simulink model "PubIfDecisionLSM_MDL"  (R2020b)
settings: configuration reference "DspaceConfig" (kept outside this file)
PostLoadFcn:
  | if any(exist('dsrtsu_mdlpostloadfcn', 'file') ~= 0), dsrtsu_mdlpostloadfcn('Execute', bdroot); end
InitFcn:
  | , if any(exist('rtifpga_mdlclblib', 'file') ~= 0), rtifpga_mdlclblib('Init', bdroot); end,
  | , if any(exist('dsmpb_private', 'file') ~= 0), dsmpb_private('dsmpb_mdlclblib', 'Init', bdroot); end,
values from neighbouring files (symbols this model uses):
  P_LSM_ALC_Enable = 0.0    [LSM_Parameter.sldd]
  P_LSM_AwayEdge_offset = 0.1    [LSM_Parameter.sldd]
  P_LSM_CentValidErr = 1.0    [LSM_Parameter.sldd]
  P_LSM_DOP_C0_EN_Limit = 0.8    [LSM_Parameter.sldd]
  P_LSM_DOP_C0_out_Limit = 2.0    [LSM_Parameter.sldd]
  P_LSM_DOP_C1_EN_Limit : value not decoded    [LSM_Parameter.sldd]
  P_LSM_DOP_C1_out_Limit : value not decoded    [LSM_Parameter.sldd]
  P_LSM_DOP_C1AndC2_Lim_X : value not decoded    [LSM_Parameter.sldd]
  P_LSM_DOP_C2_EN_Limit : value not decoded    [LSM_Parameter.sldd]
  P_LSM_DOP_C2_out_Limit : value not decoded    [LSM_Parameter.sldd]
  P_LSM_DOP_In_Pre2Dop_Dis = 1.0    [LSM_Parameter.sldd]
  P_LSM_DOP_Out_Pre2Dop_Dis = 2.0    [LSM_Parameter.sldd]
  P_LSM_DOP_PreDis_X : value not decoded    [LSM_Parameter.sldd]
  P_LSM_DOP_PreDis_Y : value not decoded    [LSM_Parameter.sldd]
  P_LSM_DOPEnableSW = 1.0    [LSM_Parameter.sldd]
  P_LSM_DOPValid_CheckTime = 0.06    [LSM_Parameter.sldd]
  P_LSM_DoubleLine_Curr2Cent_Dislimit = 0.5    [LSM_Parameter.sldd]
  P_LSM_DoubleLine_Dop2Cent_Dislimit = 0.5    [LSM_Parameter.sldd]
  P_LSM_DoubleLine_DOPOut_C1 : value not decoded    [LSM_Parameter.sldd]
  P_LSM_DoubleLine_Pre2Cent_Dislimit = 1.0    [LSM_Parameter.sldd]
  P_LSM_Error_Limit = 0.5    [LSM_Parameter.sldd]
  P_LSM_IFV2CenterAxis = 0.0    [LSM_Parameter.sldd]
  P_LSM_IFV2RearAxis = 0.0    [LSM_Parameter.sldd]
  P_LSM_Line2Edge_limit = 0.5    [LSM_Parameter.sldd]
  P_LSM_Line_Error = 0.1    [LSM_Parameter.sldd]
  P_LSM_LineSTD_Limit = 0.15    [LSM_Parameter.sldd]
  P_LSM_NOH_Switch = 0.0    [LSM_Parameter.sldd]
  P_LSM_OTL_C0_Factor = 1.0    [LSM_Parameter.sldd]
  P_LSM_OTL_C1_Factor = 0.5    [LSM_Parameter.sldd]
  P_LSM_OTL_C2_Factor = 0.5    [LSM_Parameter.sldd]
  P_LSM_Pre2OnlyLineDis = 5.0    [LSM_Parameter.sldd]
  P_LSM_Pre_t = 0.0    [LSM_Parameter.sldd]
  P_LSM_SingleLine_Cent2Edge_Dislimit = 100.0    [LSM_Parameter.sldd]
  P_LSM_SingleLine_Curr2Cent_Dislimit = 0.2    [LSM_Parameter.sldd]
  P_LSM_SingleLine_Dop2Cent_Dislimit = 0.2    [LSM_Parameter.sldd]
  P_LSM_SingleLine_DOPOut_C1 : value not decoded    [LSM_Parameter.sldd]
  P_LSM_SingleLine_Pre2Cent_Dislimit = 0.5    [LSM_Parameter.sldd]
  P_LSM_TJALimitSpd = 60.0    [LSM_Parameter.sldd]
undefined symbols (not defined in the file or in its folder): P_lCS_IFV2CenterAxis, P_LCS_IFV2RearAxis, P_LSM_EntryEdge_offset, P_LSM_EntryLnChngEnSwitch, P_LSM_EntryVanishDis, P_LSM_LinetLostTime, P_LSM_LineWijCal_C12, P_LSM_LineWijCal_C13, P_LSM_MapValid_ErrorSwitch, P_LSM_PosLineLcFac, P_LSM_SpdLim_Stub_Spd, P_LSM_SpdLim_StubLength, P_LSM_SpdTurnAlarm
libraries: simulink x324, TrueDurationTime x11
(part 23 of 25)

== matlab function PubIfDecisionLSM_MDL/Subsystem1/TargetLineCalc_20ms2/TargetLineCalc/TypeConf1/RoadWidthCalc1 ==
  data: LeftType input uint8 size=1; RightType input uint8 size=1; Cnt1K1 input uint8 size=1; Cnt2K1 input uint8 size=1; LeftEn output boolean size=1; RightEn output boolean size=1; Cnt1 output uint8 size=1; Cnt2 output uint8 size=1
function [LeftEn,RightEn,Cnt1,Cnt2] = Delay(LeftType,RightType,Cnt1K1,Cnt2K1)
Cnt1 = max(Cnt1K1 - uint8(1),uint8(0));
Cnt2 = max(Cnt2K1 - uint8(1),uint8(0));
if LeftType~=2 && LeftType~=4 && LeftType~=6 && LeftType~=20
   Cnt1 = uint8(10); 
end
if RightType~=2 && RightType~=4 && RightType~=6 && RightType~=20
   Cnt2 = uint8(10); 
end

if Cnt1>0
    LeftEn = false;
else
    LeftEn = true;
end

if Cnt2>0
    RightEn = false;
else
    RightEn = true;
end
end

== matlab function PubIfDecisionLSM_MDL/Subsystem1/TargetLineCalc_20ms2/TargetLineCalc/VehStation ==
  data: VisLineConf input uint8; LeftMostLane output boolean; VisLineA0 input single; VisLineType input uint8; VisEdgeConf input uint8; VisEdgeA0 input single; RightMostLane output boolean; VisLineColor input
function [LeftMostLane,RightMostLane] = fcn(VisLineConf,VisLineA0,VisLineType,VisEdgeConf,VisEdgeA0,VisLineColor)
LeftMostLane = false;
RightMostLane = false;
% SingleLane = false;
if (VisLineConf(2)>0&&VisEdgeConf(1)>0&&VisLineType(1)==1&&abs(VisLineA0(2)-VisEdgeA0(1))<5)||VisLineColor(1)==2
    LeftMostLane = true;
elseif (VisLineConf(3)>0&&VisEdgeConf(2)>0&&VisLineType(2)==1&&abs(VisLineA0(3)-VisEdgeA0(2))<5)||VisLineColor(2)==2
    RightMostLane = true;
end

== matlab function PubIfDecisionLSM_MDL/Subsystem1/TargetLineCalc_20ms2/TargetLineCalc/VisLineFilter1 ==
  data: tCycle input single size=1; vRef input; OTLineValid input boolean size=1; aOTL input single size=1; bOTL input single size=1; cOTL input single size=1; dOTL input single size=1; R input single size=1; LineUpdate input boolean size=1; dDeltaX input single size=1; dDeltaY input single size=1; CosOfPsi input single size=1; SinOfPsi input single size=1; LineValidK1 input boolean size=1; A3K1 input single size=1; A2K1 input single size=1; A1K1 input single size=1; A0K1 input single size=1; RangeK1 input single size=1; tLostK1 input single size=1; LineValid output boolean size=1; A3 output single size=1; A2 output single size=1; A1 output single size=1; A0 output single size=1; Range output single size=1; tLost output single size=1
function [LineValid,A3,A2,A1,A0,Range,tLost] = ...
    VisFilter(tCycle,vRef,OTLineValid,aOTL,bOTL,cOTL,dOTL,R,LineUpdate,...
    dDeltaX,dDeltaY,CosOfPsi,SinOfPsi,...
    LineValidK1,A3K1,A2K1,A1K1,A0K1,RangeK1,tLostK1)

if (OTLineValid==true)&&(LineUpdate==true)
    LineValid = true;
    A3 = aOTL;
    A2 = bOTL;
    A1 = cOTL;
    A0 = dOTL;
    Range = R;
%     if Range<RangeK1
%         Range = RangeK1 - vRef*tCycle;
%     end
    tLost = single(0);
else
    tLost = min(tLostK1 + tCycle,single(10));
    if (LineValidK1==true)&&(tLost<1)
        xi = [0;0.25*RangeK1;0.5*RangeK1;RangeK1];
        yi = A3K1*xi.^3 + A2K1*xi.^2 + A1K1*xi + A0K1;
        t_dx = xi-dDeltaX;
        t_dy = yi-dDeltaY;
        TmpX = t_dx*CosOfPsi+t_dy*SinOfPsi;
        TmpY = -t_dx*SinOfPsi+t_dy*CosOfPsi;
        [A3,A2,A1,A0] = pl(TmpX,TmpY);
        LineValid = true;
        Range = RangeK1 - vRef*tCycle;
        if Range<1
            LineValid = false;
        end
    else
        LineValid = false;
        A3 = single(0);
        A2 = single(0);
        A1 = single(0);
        A0 = single(0);
        Range = single(0);
    end
end

== matlab function PubIfDecisionLSM_MDL/Subsystem1/TargetLineCalc_20ms2/TargetLineCalc/VisLineFilter2 ==
  data: P_LSM_LinetLostTime input; tF input single size=1; DevValid output boolean size=4; DevAngle output single size=4; DevDis output single size=4; tCycle input single size=1; VisLineConf input uint8 size=4; VisLineReliable input single; a3 input single size=4; a2 input single size=4; a1 input single size=4; a0 input single size=4; R input single size=4; LineUpdate input boolean size=1; dDeltaX input single size=1; dDeltaY input single size=1; CosOfPsi input single size=1; SinOfPsi input single size=1; vRef input single size=1; Lowlimit input single; RoadWidth input single size=1; LeftLineChange input boolean size=1; RightLineChange input boolean size=1; LineConfK1 input uint8 size=4; LineReliableK1 input single; A3K1 input single size=4; A2K1 input single size=4; A1K1 input single size=4; A0K1 input single size=4; RangeK1 input single size=4; tLostK1 input single size=4; LineConf output uint8 size=4; LineReliable output single; A3 output single size=4; A2 output single size=4; A1 output single size=4; A0 output single size=4; Range output single size=4; tLost output single size=4; Avail_timeK1 input single; Avail_disK1 input single; Avail_time output single; Avail_dis output single; fix_timeK1 input; FaultK1 input; fix_time output; Fault output
    function [DevValid,DevAngle,DevDis,LineConf,LineReliable,A3,A2,A1,A0,Range,tLost,Avail_time,Avail_dis,fix_time,Fault] = ...
    VisFilter(P_LSM_LinetLostTime,tF,tCycle,VisLineConf,VisLineReliable,a3,a2,a1,a0,R,LineUpdate,...
    dDeltaX,dDeltaY,CosOfPsi,SinOfPsi,vRef,Lowlimit,RoadWidth,LeftLineChange,RightLineChange,...
    LineConfK1, LineReliableK1,A3K1,A2K1,A1K1,A0K1,RangeK1,tLostK1,Avail_timeK1,Avail_disK1,fix_timeK1,FaultK1)

LineConf = uint8(zeros(4,1));
LineReliable = single(zeros(4,1));
A3 = single(zeros(4,1));
A2 = single(zeros(4,1));
A1 = single(zeros(4,1));
A0 = single(zeros(4,1));
Range = single(zeros(4,1));
tLost = single(zeros(4,1));

Line_std = single(zeros(4,1));
Avail_time = Avail_timeK1;
Avail_dis = Avail_disK1;
fix_time = fix_timeK1;
Fault = FaultK1;

DevValid = false(4,1);
DevAngle = single(zeros(4,1));
DevDis = single(zeros(4,1));

for i=1:4
    if  (LineUpdate==true)&&(VisLineConf(i)>0)&&VisLineReliable(i)>0.01
        LineConf(i) = VisLineConf(i);
        LineReliable(i) = VisLineReliable(i);
        A3(i) = a3(i);
        A2(i) = a2(i);
        A1(i) = a1(i);
        A0(i) = a0(i);
        Range(i) = R(i);
        if Range(i)<RangeK1(i)
            Range(i) = RangeK1(i) - vRef*tCycle;
        end
        tLost(i) = single(0);
        
        if LineConfK1(i)>0
            DevValid(i) = true;
            t_Dist = max(single(15),vRef*1.8);
            xi = [0.05*t_Dist;0.3*t_Dist;0.6*t_Dist;t_Dist];
            yi = A3K1(i)*xi.^3 + A2K1(i)*xi.^2 + A1K1(i)*xi + A0K1(i);
            t_dx = xi-dDeltaX;
            t_dy = yi-dDeltaY;
            TmpX = t_dx*CosOfPsi+t_dy*SinOfPsi;
            TmpY = -t_dx*SinOfPsi+t_dy*CosOfPsi;
            [t3,t2,t1,t0] = pl(TmpX,TmpY);
            
            DevAngle(i) = 57.3*(atan(A1(i)) - atan(t1));
            DevDis(i) = (A0(i) - t0)/sqrt(A1(i)^2 + single(1));
            
            if (abs(DevAngle(i))<3)&&(abs(DevDis(i))<0.06)
                tFilter = 0.05/tF;
                A3(i) = tFilter*(A3(i) - t3) + t3;
                A2(i) = tFilter*(A2(i) - t2) + t2;
                A1(i) = tFilter*(A1(i) - t1) + t1;
                A0(i) = tFilter*(A0(i) - t0) + t0;
            end
        end
    else
        tLost(i) = min(tLostK1(i) + tCycle,single(10));
        if (LineConfK1(i)>0)&&(tLost(i)<P_LSM_LinetLostTime)&&vRef>1.8
            xi = [0.5*vRef;(0.5*vRef+0.25*RangeK1(i));(0.5*vRef+0.5*RangeK1(i));(0.5*vRef+RangeK1(i))];
            yi = A3K1(i)*xi.^3 + A2K1(i)*xi.^2 + A1K1(i)*xi + A0K1(i);
            t_dx = xi-dDeltaX;
            t_dy = yi-dDeltaY;
            TmpX = t_dx*CosOfPsi+t_dy*SinOfPsi;
            TmpY = -t_dx*SinOfPsi+t_dy*CosOfPsi;
            [A3(i),A2(i),A1(i),A0(i)] = pl(TmpX,TmpY);
            LineConf(i) = LineConfK1(i);
            LineReliable(i) = LineReliableK1(i);
            Range(i) = RangeK1(i) - 0.5*vRef*tCycle;
            if Range(i)<5
                LineConf(i) = uint8(0);
            end
        elseif (LineConfK1(i)>0)&&vRef<=1.8
            xi = [0.5*vRef;(0.5*vRef+0.25*RangeK1(i));(0.5*vRef+0.5*RangeK1(i));(0.5*vRef+RangeK1(i))];
            yi = A3K1(i)*xi.^3 + A2K1(i)*xi.^2 + A1K1(i)*xi + A0K1(i);
            t_dx = xi-dDeltaX;
            t_dy = yi-dDeltaY;
            TmpX = t_dx*CosOfPsi+t_dy*SinOfPsi;
            TmpY = -t_dx*SinOfPsi+t_dy*CosOfPsi;
            [A3(i),A2(i),A1(i),A0(i)] = pl(TmpX,TmpY);
            LineConf(i) = LineConfK1(i);
            LineReliable(i) = LineReliableK1(i);
            Range(i) = max(5,RangeK1(i));
        end
    end
end
%%  车道线校验
if LeftLineChange
    Avail_time = [single(0);Avail_timeK1(1)+tCycle;Avail_timeK1(2)+tCycle;Avail_timeK1(3)+tCycle];
    Avail_dis = [single(0);Avail_disK1(1)+tCycle*vRef;Avail_disK1(2)+tCycle*vRef;Avail_disK1(3)+tCycle*vRef];  
elseif RightLineChange
    Avail_time = [Avail_timeK1(2)+tCycle;Avail_timeK1(3)+tCycle;Avail_timeK1(4)+tCycle;single(0)];
    Avail_dis = [Avail_disK1(2)+tCycle*vRef;Avail_disK1(3)+tCycle*vRef;Avail_disK1(4)+tCycle*vRef;single(0)];
else
    for i = 1:4
        if  LineConf(i)>0
            t_Dist = max(single(15),5*vRef);
            xi = [0.05*t_Dist;0.6*t_Dist;0.8*t_Dist;t_Dist];
            yi = A3K1(i)*xi.^3 + A2K1(i)*xi.^2 + A1K1(i)*xi + A0K1(i);
            t_dx = xi-dDeltaX;
            y = A3(i)*t_dx.^3+A2(i)*t_dx.^2+A1(i)*t_dx+A0(i);
            Error = y - yi;
            Line_std(i) = std(Error);
            if Line_std(i)<Lowlimit
                Avail_time(i) = Avail_timeK1(i)+tCycle;
                Avail_dis(i) = Avail_disK1(i)+tCycle*vRef;
            else
                Avail_time(i) = single(0);
                Avail_dis(i) = single(0);
            end
%             if Avail_time(i)>6&&Avail_dis(i)>60
%                 Fault(i) = false;
%             end
%             if Fault(i)==true
%                 fix_time(i) = fix_timeK1(i)+tCycle;
%                 xi = [0.5*vRef;(0.5*vRef+0.25*RangeK1(i));(0.5*vRef+0.5*RangeK1(i));(0.5*vRef+RangeK1(i))];
%                 yi = A3K1(i)*xi.^3 + A2K1(i)*xi.^2 + A1K1(i)*xi + A0K1(i);
%                 t_dx = xi-dDeltaX;
%                 t_dy = yi-dDeltaY;
%                 TmpX = t_dx*CosOfPsi+t_dy*SinOfPsi;
%                 TmpY = -t_dx*SinOfPsi+t_dy*CosOfPsi;
%                 [A3(i),A2(i),A1(i),A0(i)] = pl(TmpX,TmpY);
%                 LineConf(i) = LineConfK1(i);
%                 LineReliable(i) = LineReliableK1(i);
%                 Range(i) = RangeK1(i) - 0.5*vRef*tCycle;
%                 if Range(i)<10||fix_time(i)>2
%                     LineConf(i) = uint8(0);
%                 end
%             else
%                 fix_time(i) = single(0);
%             end
        elseif LineConf(i)==0
            Avail_time(i) = single(0);
            Avail_dis(i) = single(0);
        end
    end
end
Avail_time = min(Avail_time,single(10));
Avail_dis = min(Avail_dis,single(100));

%%   
%    When occur left-line crossing,if L2 lost,the above line offset
%    algorithm may calculate a new L2 line,but now the new L2 line have
%    became L3 line ,so it lead to L2 line and L3 line are the same
if (LeftLineChange||RightLineChange) && VisLineConf(2)==0                       
    A3(2) = A3(3);
    A2(2) = A2(3);
    A1(2) = A1(3);
    A0(2) = A0(3)+RoadWidth*sqrt(1+A1(3)*A1(3));
    LineConf(2) = LineConf(3);
    LineReliable(2) = LineReliable(3);
    Range(2) = Range(3);
elseif  (LeftLineChange||RightLineChange) && VisLineConf(3)==0
    A3(3) = A3(2);
    A2(3) = A2(2);
    A1(3) = A1(2);
    A0(3) = A0(2)-RoadWidth*sqrt(1+A1(2)*A1(2));
    LineConf(3) = LineConf(2);
    LineReliable(3) = LineReliable(2);
    Range(3) = Range(2);
end

== matlab function PubIfDecisionLSM_MDL/Subsystem1/TargetLineCalc_20ms2/TargetLineCalc/VisLineFilter4 ==
  data: EdgeConf output uint8 size=2; EdgeReliable output single; EdgeA3 output single size=2; EdgeA2 output single size=2; EdgeA1 output single size=2; EdgeA0 output single size=2; tCycle input single size=1; VisEdgeConf input uint8 size=2; VisEdgeReliable input single; a3 input single size=2; a2 input single size=2; a1 input single size=2; a0 input single size=2; R input single size=2; LineUpdate input boolean size=1; dDeltaX input single size=1; dDeltaY input single size=1; CosOfPsi input single size=1; SinOfPsi input single size=1; vRef input single size=1; EdgeConfK1 input uint8 size=2; EdgeReliableK1 input single; EdgeA3K1 input single size=2; EdgeA2K1 input single size=2; EdgeA1K1 input single size=2; EdgeA0K1 input single size=2; EdgeRangeK1 input single size=2; EdgetLostK1 input single size=2; EdgeRange output single size=2; EdgetLost output single size=2; Avail_timeK1 input single; Avail_disK1 input single; Avail_time output single; Avail_dis output single
function [EdgeConf,EdgeReliable,EdgeA3,EdgeA2,EdgeA1,EdgeA0,EdgeRange,EdgetLost,Avail_time,Avail_dis] = ...
    VisFilter(tCycle,VisEdgeConf,VisEdgeReliable,a3,a2,a1,a0,R,LineUpdate,...
    dDeltaX,dDeltaY,CosOfPsi,SinOfPsi,vRef,EdgeConfK1,EdgeReliableK1,EdgeA3K1,...
    EdgeA2K1,EdgeA1K1,EdgeA0K1,EdgeRangeK1,EdgetLostK1,Avail_timeK1,Avail_disK1)

EdgeConf = uint8(zeros(2,1));
EdgeReliable = single(zeros(2,1));
EdgeA3 = single(zeros(2,1));
EdgeA2 = single(zeros(2,1));
EdgeA1 = single(zeros(2,1));
EdgeA0 = single(zeros(2,1));
EdgeRange = single(zeros(2,1));
EdgetLost = single(zeros(2,1));
Line_std = single(zeros(2,1));
Avail_time = Avail_timeK1;
Avail_dis = Avail_disK1;

for i=1:2
    if (VisEdgeConf(i)>0)&&(LineUpdate==true)
        EdgeConf(i) = VisEdgeConf(i);
        EdgeReliable(i) = VisEdgeReliable(i);
        EdgeA3(i) = a3(i);
        EdgeA2(i) = a2(i);
        EdgeA1(i) = a1(i);
        EdgeA0(i) = a0(i);
        EdgeRange(i) = R(i);
        EdgetLost(i) = single(0);
    else
        EdgetLost(i) = min(EdgetLostK1(i) + tCycle,single(10));
        if (EdgeConfK1(i)>0)&&(EdgetLost(i)<0.3)
            xi = [0.5*vRef;(0.5*vRef+0.25*EdgeRangeK1(i));(0.5*vRef+0.5*EdgeRangeK1(i));(0.5*vRef+EdgeRangeK1(i))];
            yi = EdgeA3K1(i)*xi.^3 + EdgeA2K1(i)*xi.^2 + EdgeA1K1(i)*xi + EdgeA0K1(i);
            t_dx = xi-dDeltaX;
            t_dy = yi-dDeltaY;
            TmpX = t_dx*CosOfPsi+t_dy*SinOfPsi;
            TmpY = -t_dx*SinOfPsi+t_dy*CosOfPsi;
            [EdgeA3(i),EdgeA2(i),EdgeA1(i),EdgeA0(i)] = pl(TmpX,TmpY);
            EdgeConf(i) = EdgeConfK1(i);
            EdgeReliable(i) = EdgeReliableK1(i);
            EdgeRange(i) = EdgeRangeK1(i) - 0.25*vRef*tCycle;
            
            if EdgeRange(i)<5
                EdgeConf(i) = uint8(0);
            end
            
        else
            EdgeConf(i) = uint8(0);
            EdgeReliable(i) = single(0);
            EdgeA3(i) = single(0);
            EdgeA2(i) = single(0);
            EdgeA1(i) = single(0);
            EdgeA0(i) = single(0);
            EdgeRange(i) = single(0);
        end
    end
end
%%  边界线校验
for i = 1:2
    if EdgeConf(i)>0
        t_Dist = max(single(15),3*vRef);
        xi = [0.05*t_Dist;0.6*t_Dist;0.8*t_Dist;t_Dist];
        yi = EdgeA3K1(i)*xi.^3 + EdgeA2K1(i)*xi.^2 + EdgeA1K1(i)*xi + EdgeA0K1(i);
        t_dx = xi-dDeltaX;
        y = EdgeA3(i)*t_dx.^3+EdgeA2(i)*t_dx.^2+EdgeA1(i)*t_dx+EdgeA0(i);
        Error = y - yi;
        Line_std(i) = std(Error);
        if Line_std(i)<0.15
            Avail_time(i) = Avail_timeK1(i)+tCycle;
            Avail_dis(i) = Avail_disK1(i)+tCycle*vRef;
        else
            Avail_time(i) = single(0);
            Avail_dis(i) = single(0);
        end
    elseif EdgeConf(i)==0
        Avail_time(i) = single(0);
        Avail_dis(i) = single(0);
    end
end

== matlab function PubIfDecisionLSM_MDL/Subsystem1/TargetLineCalc_20ms2/TargetLineCalc/YBranchRi ==
  data: LineUpdate input boolean size=1; RightOffset_b input boolean size=1; vRef input single size=1; RoadWidth input single size=1; A3 input single size=4; A2 input single size=4; A1 input single size=4; A0 input single size=4; Conf input uint8 size=4; Reliable input; DistK1 input single size=1; YBranch_b output boolean size=1; YBranchRi_b output boolean size=1; Dist output single size=1; DistRiK1 input single size=1; DistRi output single size=1
function [YBranch_b,YBranchRi_b,Dist,DistRi] =...
    fcn(LineUpdate,RightOffset_b,vRef,RoadWidth,A3,A2,A1,A0,Conf,Reliable,DistK1,DistRiK1)
%%  判断本车道40米处是否边宽变窄，或者右侧出现分叉车道
Dist = max(DistK1 - 0.02*vRef,single(0));
DistRi = max(DistRiK1 - 0.02*vRef,single(0));
if RightOffset_b
    Dist = DistRi;
    DistRi = single(0);
end
LConf = uint8(0);
RConf = uint8(0);
RRConf = uint8(0);
LA3 = A3(2);
LA2 = A2(2);
LA1 = A1(2); 
LA0 = A0(2);
if Reliable(2)>=0.9
LConf = Conf(2);
end

RA3 = A3(3);
RA2 = A2(3);
RA1 = A1(3); 
RA0 = A0(3);
if Reliable(3)>=0.9
RConf = Conf(3);
end

RRA3 = A3(4);
RRA2 = A2(4);
RRA1 = A1(4); 
RRA0 = A0(4);
if Reliable(4)>=0.9
RRConf = Conf(4);
end

if (LConf>0)&&(RConf>0)&&(LineUpdate)&&abs(LA2)<0.0005&&abs(RA2)<0.0005
    dy0 = (LA0 - RA0)/sqrt(LA1^2 +single(1));
    dy40L = 64000*LA3 + 1600*LA2 + 40*LA1 + LA0;
    dy40R = 64000*RA3 + 1600*RA2 + 40*RA1 + RA0;
    K40 = 3*LA3*1600 + 2*LA2*40 + LA1;
    dy40 = (dy40L - dy40R)/sqrt(K40^2 +single(1));
    if (dy0 - dy40<-0.5)&&(RoadWidth>2.5)&&(RoadWidth<4.2)
        Dist = single(80);
    end
end

if Dist>0
    YBranch_b = true;
else
    YBranch_b = false;
end

if (RConf>0)&&(RRConf>0)&&(LineUpdate)
    dy0 = (RA0 - RRA0)/sqrt(RA1^2 + single(1));
    dy40L = 64000*RA3 + 1600*RA2 + 40*RA1 + RA0;
    dy40R = 64000*RRA3 + 1600*RRA2 + 40*RRA1 + RRA0;
    K40 = 3*RA3*1600 + 2*RA2*40 + RA1;
    dy40 = (dy40L - dy40R)/sqrt(K40^2 + single(1));
    if (vRef>15)&&(abs(dy0 - dy40)>1.0)&&(RoadWidth>2.5)&&(RoadWidth<4.2)
        DistRi = single(80);
    end
end

if DistRi>0
    YBranchRi_b = true;
else
    YBranchRi_b = false;
end

== matlab function PubIfDecisionLSM_MDL/Subsystem1/TargetLineCalc_20ms/TargetLineCalc/TJA2NOA ==
  data: TJALineValid input boolean size=1; HWALineValid output boolean size=1; TJALineA3 input single size=1; TJALineA2 input single size=1; TJALineA1 input single size=1; TJALineA0 input single size=1; TJALineRange input single size=1; HWALineC3 output single size=1; HWALineC2 output single size=1; HWALineC1 output single size=1; HWALineC0 output single size=1; HWARange output single size=1
function [HWALineValid,HWALineC3,HWALineC2,HWALineC1,HWALineC0,HWARange] =...
    fcn(TJALineValid,TJALineA3,TJALineA2,...
    TJALineA1,TJALineA0,TJALineRange)
HWALineValid = TJALineValid;
HWALineC3 = TJALineA3;
HWALineC2 = TJALineA2;
HWALineC1 = TJALineA1;
HWALineC0 = TJALineA0;
HWARange = TJALineRange;

== matlab function PubIfDecisionLSM_MDL/Subsystem1/TargetLineCalc_20ms/TargetLineCalc/TypeConf/MATLAB Function ==
  data: update input; LeftType output uint8 size=1; LeftType_en input uint8 size=1; LeftDLMType_en input uint8 size=1; LeftDECELType_en input uint8; RightType_en input uint8 size=1; RightDLMType_en input uint8 size=1; RightDECELType_en input uint8; LeftColor_en input uint8; LLeftType_en input uint8; LeftTypeK1 input uint8 size=1; LeftDLMTypeK1 input uint8 size=1; LeftDECELTypeK1 input uint8; RightTypeK1 input uint8 size=1; RightDLMTypeK1 input uint8 size=1; LeftDLMType output uint8 size=1; LeftDECELType output; RightType output uint8 size=1; RightDLMType output uint8 size=1; RightDECELTypeK1 input uint8; RightDECELType output; LeftColor_enK1 input uint8; LLeftType_enK1 input uint8; LeftColor output; LLeftType output
function [LeftType,LeftDLMType,LeftDECELType,RightType,RightDLMType,RightDECELType,LeftColor,LLeftType] = ...
    fcn(update,LeftType_en,LeftDLMType_en,LeftDECELType_en,RightType_en,RightDLMType_en,RightDECELType_en,LeftColor_en,LLeftType_en,...
        LeftTypeK1,LeftDLMTypeK1,LeftDECELTypeK1,RightTypeK1,RightDLMTypeK1,RightDECELTypeK1,LeftColor_enK1,LLeftType_enK1)
if update
    LeftType = LeftType_en;
    LeftDLMType = LeftDLMType_en;
    LeftDECELType = LeftDECELType_en;
    RightType = RightType_en;
    RightDLMType = RightDLMType_en;
    RightDECELType = RightDECELType_en;
    LeftColor = LeftColor_en;
    LLeftType = LLeftType_en;
else
    LeftType = LeftTypeK1;
    LeftDLMType = LeftDLMTypeK1;
    LeftDECELType = LeftDECELTypeK1;
    RightType = RightTypeK1;
    RightDLMType = RightDLMTypeK1;
    RightDECELType = RightDECELTypeK1;
    LeftColor = LeftColor_enK1;
    LLeftType = LLeftType_enK1;
end

== matlab function PubIfDecisionLSM_MDL/Subsystem1/TargetLineCalc_20ms/TargetLineCalc/TypeConf/RoadWidthCalc1 ==
  data: LeftType input uint8 size=1; LeftDLMType input; LeftDECELType input; RightType input uint8 size=1; RightDLMType input; RightDECELType input; Cnt1K1 input uint8 size=1; Cnt2K1 input uint8 size=1; LeftEn output boolean size=1; RightEn output boolean size=1; Cnt1 output uint8 size=1; Cnt2 output uint8 size=1
function [LeftEn,RightEn,Cnt1,Cnt2] = Delay(LeftType,LeftDLMType,LeftDECELType,RightType,RightDLMType,RightDECELType,Cnt1K1,Cnt2K1)
Cnt1 = max(Cnt1K1 - uint8(1),uint8(0));
Cnt2 = max(Cnt2K1 - uint8(1),uint8(0));
if LeftType==1||LeftType==6||(LeftType==3&&(LeftDLMType~=2||LeftDLMType~=4))||(LeftType==5&&(LeftDECELType~=2))
   Cnt1 = uint8(10); 
end
if RightType==1||RightType==6||(RightType==3&&(RightDLMType~=2||RightDLMType~=4))||(RightType==5&&(RightDECELType~=2))
   Cnt2 = uint8(10); 
end

if Cnt1>0
    LeftEn = false;
else
    LeftEn = true;
end

if Cnt2>0
    RightEn = false;
else
    RightEn = true;
end
end

== matlab function PubIfDecisionLSM_MDL/Subsystem1/TargetLineCalc_20ms/TargetLineCalc/TypeConf1/RoadWidthCalc1 ==
  data: LeftType input uint8 size=1; RightType input uint8 size=1; Cnt1K1 input uint8 size=1; Cnt2K1 input uint8 size=1; LeftEn output boolean size=1; RightEn output boolean size=1; Cnt1 output uint8 size=1; Cnt2 output uint8 size=1
function [LeftEn,RightEn,Cnt1,Cnt2] = Delay(LeftType,RightType,Cnt1K1,Cnt2K1)
Cnt1 = max(Cnt1K1 - uint8(1),uint8(0));
Cnt2 = max(Cnt2K1 - uint8(1),uint8(0));
if LeftType~=2 || LeftType~=4 || LeftType~=6
   Cnt1 = uint8(10); 
end
if RightType~=2 || RightType~=4 || RightType~=6
   Cnt2 = uint8(10); 
end

if Cnt1>0
    LeftEn = false;
else
    LeftEn = true;
end

if Cnt2>0
    RightEn = false;
else
    RightEn = true;
end
end

== matlab function PubIfDecisionLSM_MDL/Subsystem1/TargetLineCalc_20ms/TargetLineCalc/VehStation ==
  data: VisLineConf input uint8; LeftMostLane output boolean; VisLineA0 input single; VisLineType input uint8; VisEdgeConf input uint8; VisEdgeA0 input single; RightMostLane output boolean; VisLineColor input
function [LeftMostLane,RightMostLane] = fcn(VisLineConf,VisLineA0,VisLineType,VisEdgeConf,VisEdgeA0,VisLineColor)
LeftMostLane = false;
RightMostLane = false;
% SingleLane = false;
if (VisLineConf(2)>0&&VisEdgeConf(1)>0&&VisLineType(1)==1&&abs(VisLineA0(2)-VisEdgeA0(1))<5)||VisLineColor(1)==2
    LeftMostLane = true;
elseif (VisLineConf(3)>0&&VisEdgeConf(2)>0&&VisLineType(2)==1&&abs(VisLineA0(3)-VisEdgeA0(2))<5)||VisLineColor(2)==2
    RightMostLane = true;
end

== matlab function PubIfDecisionLSM_MDL/Subsystem1/TargetLineCalc_20ms/TargetLineCalc/VisLineFilter1 ==
  data: tCycle input single size=1; vRef input; OTLineValid input boolean size=1; aOTL input single size=1; bOTL input single size=1; cOTL input single size=1; dOTL input single size=1; R input single size=1; LineUpdate input boolean size=1; dDeltaX input single size=1; dDeltaY input single size=1; CosOfPsi input single size=1; SinOfPsi input single size=1; LineValidK1 input boolean size=1; A3K1 input single size=1; A2K1 input single size=1; A1K1 input single size=1; A0K1 input single size=1; RangeK1 input single size=1; tLostK1 input single size=1; LineValid output boolean size=1; A3 output single size=1; A2 output single size=1; A1 output single size=1; A0 output single size=1; Range output single size=1; tLost output single size=1
function [LineValid,A3,A2,A1,A0,Range,tLost] = ...
    VisFilter(tCycle,vRef,OTLineValid,aOTL,bOTL,cOTL,dOTL,R,LineUpdate,...
    dDeltaX,dDeltaY,CosOfPsi,SinOfPsi,...
    LineValidK1,A3K1,A2K1,A1K1,A0K1,RangeK1,tLostK1)

if (OTLineValid==true)&&(LineUpdate==true)
    LineValid = true;
    A3 = aOTL;
    A2 = bOTL;
    A1 = cOTL;
    A0 = dOTL;
    Range = R;
%     if Range<RangeK1
%         Range = RangeK1 - vRef*tCycle;
%     end
    tLost = single(0);
else
    tLost = min(tLostK1 + tCycle,single(10));
    if (LineValidK1==true)&&(tLost<1)&&vRef>1.8
        xi = [0;0.25*RangeK1;0.5*RangeK1;RangeK1];
        yi = A3K1*xi.^3 + A2K1*xi.^2 + A1K1*xi + A0K1;
        t_dx = xi-dDeltaX;
        t_dy = yi-dDeltaY;
        TmpX = t_dx*CosOfPsi+t_dy*SinOfPsi;
        TmpY = -t_dx*SinOfPsi+t_dy*CosOfPsi;
        [A3,A2,A1,A0] = pl(TmpX,TmpY);
        LineValid = true;
        Range = RangeK1 - vRef*tCycle;
        if Range<1
            LineValid = false;
        end
    elseif LineValidK1==true&&vRef<=1.8
         xi = [0;0.25*RangeK1;0.5*RangeK1;RangeK1];
        yi = A3K1*xi.^3 + A2K1*xi.^2 + A1K1*xi + A0K1;
        t_dx = xi-dDeltaX;
        t_dy = yi-dDeltaY;
        TmpX = t_dx*CosOfPsi+t_dy*SinOfPsi;
        TmpY = -t_dx*SinOfPsi+t_dy*CosOfPsi;
        [A3,A2,A1,A0] = pl(TmpX,TmpY);
        LineValid = true;
        Range = max(single(5),RangeK1);
    else
        LineValid = false;
        A3 = single(0);
        A2 = single(0);
        A1 = single(0);
        A0 = single(0);
        Range = single(0);
    end
end

== matlab function PubIfDecisionLSM_MDL/Subsystem1/TargetLineCalc_20ms/TargetLineCalc/VisLineFilter2 ==
  data: tF input single size=1; DevValid output boolean size=4; DevAngle output single size=4; DevDis output single size=4; tCycle input single size=1; VisLineConf input uint8 size=4; VisLineReliable input single; a3 input single size=4; a2 input single size=4; a1 input single size=4; a0 input single size=4; R input single size=4; LineUpdate input boolean size=1; dDeltaX input single size=1; dDeltaY input single size=1; CosOfPsi input single size=1; SinOfPsi input single size=1; vRef input single size=1; Lowlimit input single; RoadWidth input single size=1; LeftLineChange input boolean size=1; RightLineChange input boolean size=1; LH1Wij input single; LH2Wij input single; LineConfK1 input uint8 size=4; LineReliableK1 input single; A3K1 input single size=4; A2K1 input single size=4; A1K1 input single size=4; A0K1 input single size=4; RangeK1 input single size=4; tLostK1 input single size=4; LineConf output uint8 size=4; LineReliable output single; A3 output single size=4; A2 output single size=4; A1 output single size=4; A0 output single size=4; Range output single size=4; tLost output single size=4; Avail_timeK1 input single; Avail_disK1 input single; Avail_time output single; Avail_dis output single; fix_timeK1 input; FaultK1 input; fix_time output; Fault output
    function [DevValid,DevAngle,DevDis,LineConf,LineReliable,A3,A2,A1,A0,Range,tLost,Avail_time,Avail_dis,fix_time,Fault] = ...
    VisFilter(tF,tCycle,VisLineConf,VisLineReliable,a3,a2,a1,a0,R,LineUpdate,...
    dDeltaX,dDeltaY,CosOfPsi,SinOfPsi,vRef,Lowlimit,RoadWidth,LeftLineChange,RightLineChange,LH1Wij,LH2Wij,...
    LineConfK1, LineReliableK1,A3K1,A2K1,A1K1,A0K1,RangeK1,tLostK1,Avail_timeK1,Avail_disK1,fix_timeK1,FaultK1)

LineConf = uint8(zeros(4,1));
LineReliable = single(zeros(4,1));
A3 = single(zeros(4,1));
A2 = single(zeros(4,1));
A1 = single(zeros(4,1));
A0 = single(zeros(4,1));
Range = single(zeros(4,1));
tLost = single(zeros(4,1));

Line_std = single(zeros(4,1));
Avail_time = Avail_timeK1;
Avail_dis = Avail_disK1;
fix_time = fix_timeK1;
Fault = FaultK1;

DevValid = false(4,1);
DevAngle = single(zeros(4,1));
DevDis = single(zeros(4,1));

for i=1:4
    if  (LineUpdate==true)&&(VisLineConf(i)>0)&&VisLineReliable(i)>0.01  
        LineConf(i) = VisLineConf(i);
        LineReliable(i) = VisLineReliable(i);
        A3(i) = a3(i);
        A2(i) = a2(i);
        A1(i) = a1(i);
        A0(i) = a0(i);
        Range(i) = R(i);
        if Range(i)<RangeK1(i)
            Range(i) = RangeK1(i) - vRef*tCycle;
        end
        tLost(i) = single(0);
        
        if LineConfK1(i)>0
            DevValid(i) = true;
            t_Dist = max(single(15),vRef*1.8);
            xi = [0.05*t_Dist;0.3*t_Dist;0.6*t_Dist;t_Dist];
            yi = A3K1(i)*xi.^3 + A2K1(i)*xi.^2 + A1K1(i)*xi + A0K1(i);
            t_dx = xi-dDeltaX;
            t_dy = yi-dDeltaY;
            TmpX = t_dx*CosOfPsi+t_dy*SinOfPsi;
            TmpY = -t_dx*SinOfPsi+t_dy*CosOfPsi;
            [t3,t2,t1,t0] = pl(TmpX,TmpY);
            
            DevAngle(i) = 57.3*(atan(A1(i)) - atan(t1));
            DevDis(i) = (A0(i) - t0)/sqrt(A1(i)^2 + single(1));
            
            if (abs(DevAngle(i))<3)&&(abs(DevDis(i))<0.06)
                tFilter = 0.05/tF;
                A3(i) = tFilter*(A3(i) - t3) + t3;
                A2(i) = tFilter*(A2(i) - t2) + t2;
                A1(i) = tFilter*(A1(i) - t1) + t1;
                A0(i) = tFilter*(A0(i) - t0) + t0;
            end
        end
    else
        tLost(i) = min(tLostK1(i) + tCycle,single(10));
        if (LineConfK1(i)>0)&&(tLost(i)<0.5)&&vRef>1.8
            xi = [0.5*vRef;(0.5*vRef+0.25*RangeK1(i));(0.5*vRef+0.5*RangeK1(i));(0.5*vRef+RangeK1(i))];
            yi = A3K1(i)*xi.^3 + A2K1(i)*xi.^2 + A1K1(i)*xi + A0K1(i);
            t_dx = xi-dDeltaX;
            t_dy = yi-dDeltaY;
            TmpX = t_dx*CosOfPsi+t_dy*SinOfPsi;
            TmpY = -t_dx*SinOfPsi+t_dy*CosOfPsi;
            [A3(i),A2(i),A1(i),A0(i)] = pl(TmpX,TmpY);
            LineConf(i) = LineConfK1(i);
            LineReliable(i) = LineReliableK1(i);
            Range(i) = RangeK1(i) - 0.5*vRef*tCycle;
            if Range(i)<5
                LineConf(i) = uint8(0);
            end
        elseif (LineConfK1(i)>0)&&vRef<=1.8
            xi = [0.5*vRef;(0.5*vRef+0.25*RangeK1(i));(0.5*vRef+0.5*RangeK1(i));(0.5*vRef+RangeK1(i))];
            yi = A3K1(i)*xi.^3 + A2K1(i)*xi.^2 + A1K1(i)*xi + A0K1(i);
            t_dx = xi-dDeltaX;
            t_dy = yi-dDeltaY;
            TmpX = t_dx*CosOfPsi+t_dy*SinOfPsi;
            TmpY = -t_dx*SinOfPsi+t_dy*CosOfPsi;
            [A3(i),A2(i),A1(i),A0(i)] = pl(TmpX,TmpY);
            LineConf(i) = LineConfK1(i);
            LineReliable(i) = LineReliableK1(i);
            Range(i) = max(5,RangeK1(i));
        end
    end
end
%%  车道线校验
if LeftLineChange
    Avail_time = [single(0);Avail_timeK1(1)+tCycle;Avail_timeK1(2)+tCycle;Avail_timeK1(3)+tCycle];
    Avail_dis = [single(0);Avail_disK1(1)+tCycle*vRef;Avail_disK1(2)+tCycle*vRef;Avail_disK1(3)+tCycle*vRef];  
elseif RightLineChange
    Avail_time = [Avail_timeK1(2)+tCycle;Avail_timeK1(3)+tCycle;Avail_timeK1(4)+tCycle;single(0)];
    Avail_dis = [Avail_disK1(2)+tCycle*vRef;Avail_disK1(3)+tCycle*vRef;Avail_disK1(4)+tCycle*vRef;single(0)];
else
    for i = 1:4
        if  LineConf(i)>0
            t_Dist = max(single(15),5*vRef);
            xi = [0.05*t_Dist;0.6*t_Dist;0.8*t_Dist;t_Dist];
            yi = A3K1(i)*xi.^3 + A2K1(i)*xi.^2 + A1K1(i)*xi + A0K1(i);
            t_dx = xi-dDeltaX;
            y = A3(i)*t_dx.^3+A2(i)*t_dx.^2+A1(i)*t_dx+A0(i);
            Error = y - yi;
            Line_std(i) = std(Error);
            if Line_std(i)<Lowlimit
                Avail_time(i) = Avail_timeK1(i)+tCycle;
                Avail_dis(i) = Avail_disK1(i)+tCycle*vRef;
            else
                Avail_time(i) = single(0);
                Avail_dis(i) = single(0);
            end
%             if Avail_time(i)>6&&Avail_dis(i)>60
%                 Fault(i) = false;
%             end
%             if Fault(i)==true
%                 fix_time(i) = fix_timeK1(i)+tCycle;
%                 xi = [0.5*vRef;(0.5*vRef+0.25*RangeK1(i));(0.5*vRef+0.5*RangeK1(i));(0.5*vRef+RangeK1(i))];
%                 yi = A3K1(i)*xi.^3 + A2K1(i)*xi.^2 + A1K1(i)*xi + A0K1(i);
%                 t_dx = xi-dDeltaX;
%                 t_dy = yi-dDeltaY;
%                 TmpX = t_dx*CosOfPsi+t_dy*SinOfPsi;
%                 TmpY = -t_dx*SinOfPsi+t_dy*CosOfPsi;
%                 [A3(i),A2(i),A1(i),A0(i)] = pl(TmpX,TmpY);
%                 LineConf(i) = LineConfK1(i);
%                 LineReliable(i) = LineReliableK1(i);
%                 Range(i) = RangeK1(i) - 0.5*vRef*tCycle;
%                 if Range(i)<10||fix_time(i)>2
%                     LineConf(i) = uint8(0);
%                 end
%             else
%                 fix_time(i) = single(0);
%             end
        elseif LineConf(i)==0
            Avail_time(i) = single(0);
            Avail_dis(i) = single(0);
        end
    end
end
Avail_time = min(Avail_time,single(10));
Avail_dis = min(Avail_dis,single(100));

%%   
%    When occur left-line crossing,if L2 lost,the above line offset
%    algorithm may calculate a new L2 line,but now the new L2 line have
%    became L3 line ,so it lead to L2 line and L3 line are the same
if (LeftLineChange||RightLineChange) && VisLineConf(2)==0                       
    A3(2) = A3(3);
    A2(2) = A2(3);
    A1(2) = A1(3);
    A0(2) = A0(3)+RoadWidth*sqrt(1+A1(3)*A1(3));
    LineConf(2) = LineConf(3);
    LineReliable(2) = LineReliable(3);
    Range(2) = Range(3);
elseif  (LeftLineChange||RightLineChange) && VisLineConf(3)==0
    A3(3) = A3(2);
    A2(3) = A2(2);
    A1(3) = A1(2);
    A0(3) = A0(2)-RoadWidth*sqrt(1+A1(2)*A1(2));
    LineConf(3) = LineConf(2);
    LineReliable(3) = LineReliable(2);
    Range(3) = Range(2);
end

== matlab function PubIfDecisionLSM_MDL/Subsystem1/TargetLineCalc_20ms/TargetLineCalc/VisLineFilter3 ==
  data: DoubleLineLost_b output; LeftOffset_b output boolean; RightOffset_b output boolean; Quality output single; tCycle input single size=1; vRef input; CentLineValid input boolean size=1; CentLineA3 input single size=1; CentLineA2 input single size=1; CentLineA1 input single size=1; CentLineA0 input single; CentLineRange input single; CentQ input single size=1; RoadWidth input; LineUpdate input boolean size=1; dDeltaX input single size=1; dDeltaY input single size=1; CosOfPsi input single size=1; SinOfPsi input single size=1; QualityK1 input single; LineValidK1 input boolean size=1; A3K1 input single size=1; A2K1 input single size=1; A1K1 input single size=1; A0K1 input single size=1; RangeK1 input single size=1; tLostK1 input single size=1; LineValid output boolean size=1; A3 output single size=1; A2 output single size=1; A1 output single size=1; A0 output single size=1; Range output single size=1; tLost output single size=1
function [DoubleLineLost_b,LeftOffset_b,RightOffset_b,Quality,LineValid,A3,A2,A1,A0,Range,tLost] = ...
    VisFilter(tCycle,vRef,CentLineValid,CentLineA3,CentLineA2,CentLineA1,CentLineA0,CentLineRange, CentQ, RoadWidth,LineUpdate,...
    dDeltaX,dDeltaY,CosOfPsi,SinOfPsi,...
    QualityK1,LineValidK1,A3K1,A2K1,A1K1,A0K1,RangeK1,tLostK1)

if (CentLineValid==true)&&(LineUpdate==true)
    LineValid = true;
    A3 = CentLineA3;
    A2 = CentLineA2;
    A1 = CentLineA1;
    A0 = CentLineA0;
    Range = CentLineRange;
    Quality=single(CentQ);
    %     if Range<RangeK1
    %         Range = RangeK1 - vRef*tCycle;
    %     end
    tLost = single(0);
else
    tLost = min(tLostK1 + tCycle,single(10));
    if (LineValidK1==true)&&(tLost<0.5)
        xi = [0;0.25*RangeK1;0.5*RangeK1;RangeK1];
        yi = A3K1*xi.^3 + A2K1*xi.^2 + A1K1*xi + A0K1;
        t_dx = xi-dDeltaX;
        t_dy = yi-dDeltaY;
        TmpX = t_dx*CosOfPsi+t_dy*SinOfPsi;
        TmpY = -t_dx*SinOfPsi+t_dy*CosOfPsi;
        [A3,A2,A1,A0] = pl(TmpX,TmpY);
        LineValid = true;
        Quality=QualityK1;
        Range = RangeK1;
        if Range<5
            LineValid = false;
        end
    else
        LineValid = false;
        A3 = single(0);
        A2 = single(0);
        A1 = single(0);
        A0 = single(0);
        Range = single(0);
        Quality=single(0);
    end
end

if (A0>0)&&(A0K1<0)&&...
        (abs(A0-A0K1)>(RoadWidth - single(1.5)))&&...
        (LineValid==true)&&(LineValidK1==true)
    LeftOffset_b = true;
else
    LeftOffset_b = false;
end
if (A0<0)&&(A0K1>0)&&...
        (abs(A0-A0K1)>(RoadWidth - single(1.5)))&&...
        (LineValid==true)&&(LineValidK1==true)
    RightOffset_b = true;
else
    RightOffset_b = false;
end


if LineValid==false
    DoubleLineLost_b = true;
else
    DoubleLineLost_b = false;
end

== matlab function PubIfDecisionLSM_MDL/Subsystem1/TargetLineCalc_20ms/TargetLineCalc/VisLineFilter4 ==
  data: EdgeConf output uint8 size=2; EdgeReliable output single; EdgeA3 output single size=2; EdgeA2 output single size=2; EdgeA1 output single size=2; EdgeA0 output single size=2; tCycle input single size=1; VisEdgeConf input uint8 size=2; VisEdgeReliable input single; a3 input single size=2; a2 input single size=2; a1 input single size=2; a0 input single size=2; R input single size=2; LineUpdate input boolean size=1; dDeltaX input single size=1; dDeltaY input single size=1; CosOfPsi input single size=1; SinOfPsi input single size=1; vRef input single size=1; EdgeConfK1 input uint8 size=2; EdgeReliableK1 input single; EdgeA3K1 input single size=2; EdgeA2K1 input single size=2; EdgeA1K1 input single size=2; EdgeA0K1 input single size=2; EdgeRangeK1 input single size=2; EdgetLostK1 input single size=2; EdgeRange output single size=2; EdgetLost output single size=2; Avail_timeK1 input single; Avail_disK1 input single; Avail_time output single; Avail_dis output single
function [EdgeConf,EdgeReliable,EdgeA3,EdgeA2,EdgeA1,EdgeA0,EdgeRange,EdgetLost,Avail_time,Avail_dis] = ...
    VisFilter(tCycle,VisEdgeConf,VisEdgeReliable,a3,a2,a1,a0,R,LineUpdate,...
    dDeltaX,dDeltaY,CosOfPsi,SinOfPsi,vRef,EdgeConfK1,EdgeReliableK1,EdgeA3K1,...
    EdgeA2K1,EdgeA1K1,EdgeA0K1,EdgeRangeK1,EdgetLostK1,Avail_timeK1,Avail_disK1)

EdgeConf = uint8(zeros(2,1));
EdgeReliable = single(zeros(2,1));
EdgeA3 = single(zeros(2,1));
EdgeA2 = single(zeros(2,1));
EdgeA1 = single(zeros(2,1));
EdgeA0 = single(zeros(2,1));
EdgeRange = single(zeros(2,1));
EdgetLost = single(zeros(2,1));
Line_std = single(zeros(2,1));
Avail_time = Avail_timeK1;
Avail_dis = Avail_disK1;

for i=1:2
    if (VisEdgeConf(i)>0)&&(LineUpdate==true)
        EdgeConf(i) = VisEdgeConf(i);
        EdgeReliable(i) = VisEdgeReliable(i);
        EdgeA3(i) = a3(i);
        EdgeA2(i) = a2(i);
        EdgeA1(i) = a1(i);
        EdgeA0(i) = a0(i);
        EdgeRange(i) = R(i);
        EdgetLost(i) = single(0);
    else
        EdgetLost(i) = min(EdgetLostK1(i) + tCycle,single(10));
        if (EdgeConfK1(i)>0)&&(EdgetLost(i)<0.3)
            xi = [0.5*vRef;(0.5*vRef+0.25*EdgeRangeK1(i));(0.5*vRef+0.5*EdgeRangeK1(i));(0.5*vRef+EdgeRangeK1(i))];
            yi = EdgeA3K1(i)*xi.^3 + EdgeA2K1(i)*xi.^2 + EdgeA1K1(i)*xi + EdgeA0K1(i);
            t_dx = xi-dDeltaX;
            t_dy = yi-dDeltaY;
            TmpX = t_dx*CosOfPsi+t_dy*SinOfPsi;
            TmpY = -t_dx*SinOfPsi+t_dy*CosOfPsi;
            [EdgeA3(i),EdgeA2(i),EdgeA1(i),EdgeA0(i)] = pl(TmpX,TmpY);
            EdgeConf(i) = EdgeConfK1(i);
            EdgeReliable(i) = EdgeReliableK1(i);
            EdgeRange(i) = EdgeRangeK1(i) - 0.25*vRef*tCycle;
            
            if EdgeRange(i)<5
                EdgeConf(i) = uint8(0);
            end
            
        else
            EdgeConf(i) = uint8(0);
            EdgeReliable(i) = single(0);
            EdgeA3(i) = single(0);
            EdgeA2(i) = single(0);
            EdgeA1(i) = single(0);
            EdgeA0(i) = single(0);
            EdgeRange(i) = single(0);
        end
    end
end
%%  边界线校验
for i = 1:2
    if EdgeConf(i)>0
        t_Dist = max(single(15),3*vRef);
        xi = [0.05*t_Dist;0.6*t_Dist;0.8*t_Dist;t_Dist];
        yi = EdgeA3K1(i)*xi.^3 + EdgeA2K1(i)*xi.^2 + EdgeA1K1(i)*xi + EdgeA0K1(i);
        t_dx = xi-dDeltaX;
        y = EdgeA3(i)*t_dx.^3+EdgeA2(i)*t_dx.^2+EdgeA1(i)*t_dx+EdgeA0(i);
        Error = y - yi;
        Line_std(i) = std(Error);
        if Line_std(i)<0.15
            Avail_time(i) = Avail_timeK1(i)+tCycle;
            Avail_dis(i) = Avail_disK1(i)+tCycle*vRef;
        else
            Avail_time(i) = single(0);
            Avail_dis(i) = single(0);
        end
    elseif EdgeConf(i)==0
        Avail_time(i) = single(0);
        Avail_dis(i) = single(0);
    end
end

== matlab function PubIfDecisionLSM_MDL/Subsystem1/TargetLineCalc_20ms/TargetLineCalc/VisLineFilter5 ==
  data: LeftOffset_b input boolean size=1; RightOffset_b input boolean; LckLock_b input boolean size=1; LckLock_bK1 input boolean size=1; CentLineValid input boolean size=1; CentLineC3 input single size=1; CentLineC2 input single; CentLineC1 input single; CentLineC0 input single; CentLineRange input single; CentLineReliable input single; LeftLineValid input boolean; LeftLineC3 input single; LeftLineC2 input single; LeftLineC1 input single; LeftLineC0 input single; LeftLineRange input single; LeftLineReliable input single; LeftLaneAvail input boolean; RightLineValid input boolean; RightLineC3 input single; RightLineC2 input single; RightLineC1 input single; RightLineC0 input single; RightLineRange input single; RightLineReliable input single; PathValid output boolean; PathA3 output single; PathA2 output single; PathA1 output single; PathA0 output single; PathRange output single; PathReliable output single; RightLaneAvail input boolean; PathLaneAvail output boolean size=3; LockIDK1 input int8; LockID output int8
function [PathValid,PathA3,PathA2,PathA1,PathA0,PathRange,PathReliable,PathLaneAvail,LockID] = ...
    VisFilter(LeftOffset_b,RightOffset_b,LckLock_b,LckLock_bK1,...
    CentLineValid,CentLineC3,CentLineC2,CentLineC1,CentLineC0,CentLineRange,CentLineReliable,...
    LeftLineValid,LeftLineC3,LeftLineC2,LeftLineC1,LeftLineC0,LeftLineRange,LeftLineReliable,LeftLaneAvail,...
    RightLineValid,RightLineC3,RightLineC2,RightLineC1,RightLineC0,RightLineRange,RightLineReliable,RightLaneAvail,LockIDK1)

PathValid = false(3,1);
PathA3 = single(zeros(3,1));
PathA2 = single(zeros(3,1));
PathA1 = single(zeros(3,1));
PathA0 = single(zeros(3,1));
PathRange = single(zeros(3,1));
PathReliable = single(zeros(3,1));
PathLaneAvail = false(3,1);

if LckLock_b
    LockID = LockIDK1;
else
    LockID = int8(0);
end

if (LckLock_b==true)&&(LckLock_bK1==true)
    if LeftOffset_b
        LockID = LockID + int8(1);
    end
    if RightOffset_b
        LockID = LockID + int8(-1);
    end
end

if LockID==int8(1)
    PathValid(2) = RightLineValid;
    PathA3(2) = RightLineC3;
    PathA2(2) = RightLineC2;
    PathA1(2) = RightLineC1;
    PathA0(2) = RightLineC0;
    PathRange(2) = RightLineRange;
    PathReliable(2) = RightLineReliable;
    PathLaneAvail(2) = true;
elseif LockID==int8(-1)
    PathValid(2) = LeftLineValid;
    PathA3(2) = LeftLineC3;
    PathA2(2) = LeftLineC2;
    PathA1(2) = LeftLineC1;
    PathA0(2) = LeftLineC0;
    PathRange(2) = LeftLineRange;
    PathReliable(2) = LeftLineReliable;
    PathLaneAvail(2) = true;
elseif LockID==int8(0)
    PathValid(1) = LeftLineValid;
    PathA3(1) = LeftLineC3;
    PathA2(1) = LeftLineC2;
    PathA1(1) = LeftLineC1;
    PathA0(1) = LeftLineC0;
    PathRange(1) = LeftLineRange;
    PathReliable(1) = LeftLineReliable;
    PathLaneAvail(1) = LeftLaneAvail;
    
    PathValid(2) = CentLineValid;
    PathA3(2) = CentLineC3;
    PathA2(2) = CentLineC2;
    PathA1(2) = CentLineC1;
    PathA0(2) = CentLineC0;
    PathRange(2) = CentLineRange;
    PathReliable(2) = CentLineReliable;
    PathLaneAvail(2) = true;
    
    PathValid(3) = RightLineValid;
    PathA3(3) = RightLineC3;
    PathA2(3) = RightLineC2;
    PathA1(3) = RightLineC1;
    PathA0(3) = RightLineC0;
    PathRange(3) = RightLineRange;
    PathReliable(3) = RightLineReliable;
    PathLaneAvail(3) = RightLaneAvail;
end

== matlab function PubIfDecisionLSM_MDL/Subsystem1/TargetLineCalc_20ms/TargetLineCalc/YBranchRi ==
  data: LineUpdate input boolean size=1; RightOffset_b input boolean size=1; vRef input single size=1; RoadWidth input single size=1; A3 input single size=4; A2 input single size=4; A1 input single size=4; A0 input single size=4; Conf input uint8 size=4; Reliable input; DistK1 input single size=1; YBranch_b output boolean size=1; YBranchRi_b output boolean size=1; Dist output single size=1; DistRiK1 input single size=1; DistRi output single size=1
function [YBranch_b,YBranchRi_b,Dist,DistRi] =...
    fcn(LineUpdate,RightOffset_b,vRef,RoadWidth,A3,A2,A1,A0,Conf,Reliable,DistK1,DistRiK1)
%%  判断本车道40米处是否边宽变窄，或者右侧出现分叉车道
Dist = max(DistK1 - 0.02*vRef,single(0));
DistRi = max(DistRiK1 - 0.02*vRef,single(0));
if RightOffset_b
    Dist = DistRi;
    DistRi = single(0);
end
LConf = uint8(0);
RConf = uint8(0);
RRConf = uint8(0);
LA3 = A3(2);
LA2 = A2(2);
LA1 = A1(2); 
LA0 = A0(2);
if Reliable(2)>=0.9
LConf = Conf(2);
end

RA3 = A3(3);
RA2 = A2(3);
RA1 = A1(3); 
RA0 = A0(3);
if Reliable(3)>=0.9
RConf = Conf(3);
end

RRA3 = A3(4);
RRA2 = A2(4);
RRA1 = A1(4); 
RRA0 = A0(4);
if Reliable(4)>=0.9
RRConf = Conf(4);
end

if (LConf>0)&&(RConf>0)&&(LineUpdate)&&abs(LA2)<0.0005&&abs(RA2)<0.0005
    dy0 = (LA0 - RA0)/sqrt(LA1^2 +single(1));
    dy40L = 64000*LA3 + 1600*LA2 + 40*LA1 + LA0;
    dy40R = 64000*RA3 + 1600*RA2 + 40*RA1 + RA0;
    K40 = 3*LA3*1600 + 2*LA2*40 + LA1;
    dy40 = (dy40L - dy40R)/sqrt(K40^2 +single(1));
    if (dy0 - dy40<-0.5)&&(RoadWidth>2.5)&&(RoadWidth<4.2)
        Dist = single(20);
    end
end

if Dist>0
    YBranch_b = true;
else
    YBranch_b = false;
end

if (RConf>0)&&(RRConf>0)&&(LineUpdate)
    dy0 = (RA0 - RRA0)/sqrt(RA1^2 + single(1));
    dy40L = 64000*RA3 + 1600*RA2 + 40*RA1 + RA0;
    dy40R = 64000*RRA3 + 1600*RRA2 + 40*RRA1 + RRA0;
    K40 = 3*RA3*1600 + 2*RA2*40 + RA1;
    dy40 = (dy40L - dy40R)/sqrt(K40^2 + single(1));
    if (vRef>15)&&(abs(dy0 - dy40)>1.0)&&(RoadWidth>2.5)&&(RoadWidth<4.2)
        DistRi = single(20);
    end
end

if DistRi>0
    YBranchRi_b = true;
else
    YBranchRi_b = false;
end
